simulink model "uvod_PID"  (R2023a)
settings: Solver=VariableStepAuto  StartTime=0.0  StopTime=40  RelTol=1e-3
values from neighbouring files (symbols this model uses):
  T = 0.01    [D1.m]    (also in D1_param.m)
libraries: simulink x1
settings Model: Creator=rapaja  LastModifiedBy=aleks
settings SolverCC: AlgebraicLoopSolver=TrustRegion
settings DebuggingCC: UnconnectedInputMsg=warning  UnconnectedOutputMsg=warning  UnconnectedLineMsg=warning
settings ModelReferenceCC: EnableRefExpFcnMdlSchedulingChecks=on

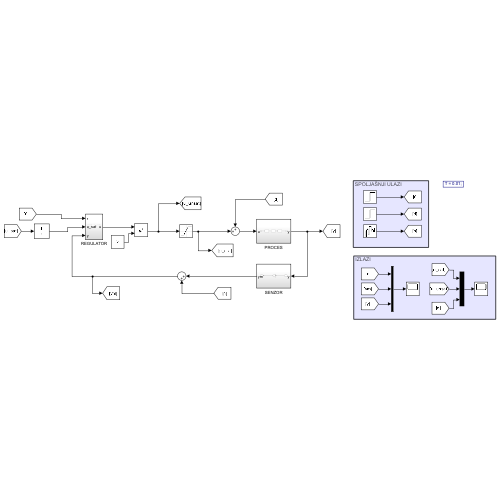
[thumbnail: Simulink's stored preview of the top-level diagram]
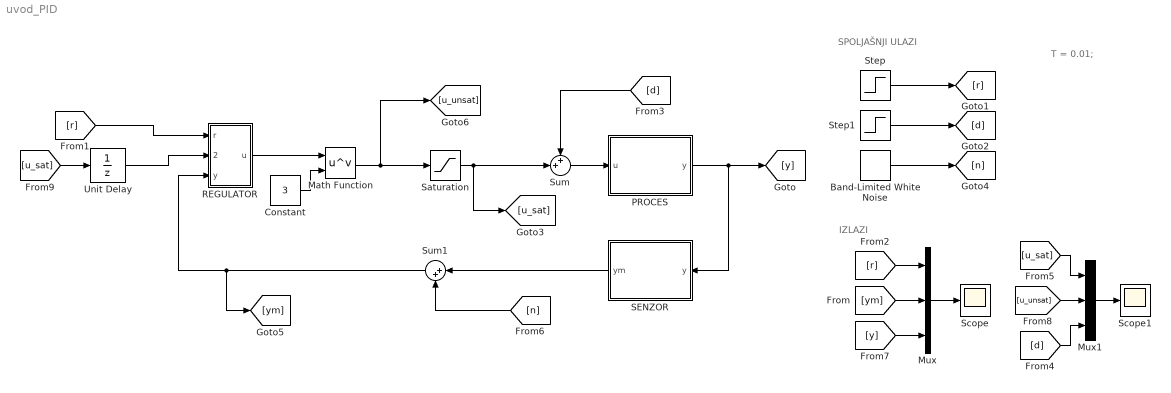
== system uvod_PID ==
  note: T = 0.01;
  note: IZLAZI
  note: SPOLJAŠNJI ULAZI
  Band-Limited White Noise : simulink/Sources/Band-Limited White Noise  Cov=[0.00001]  Ts=T  seed=[23341]
  Constant : Constant  Value=3
  Math Function : Math  Operator=pow
  Mux : Mux  Inputs=3
  Mux1 : Mux  Inputs=3
  PROCES : Subsystem
  REGULATOR : Subsystem
  SENZOR : Subsystem
  Saturation : Saturate  UpperLimit=1  LowerLimit=-1
  Scope : Scope
  Scope1 : Scope
  Step : Step  SampleTime=0
  Step1 : Step  Time=10  SampleTime=0
  Sum : Sum  Inputs=++|
  Sum1 : Sum  Inputs=|++
  Unit Delay : UnitDelay  SampleTime=-1  HasFrameUpgradeWarning=on
  wires:
  [r] -> Mux/1
  [ym] -> Mux/2
  Mux/1 -> Scope/1
  Step/1 -> [r]
  Sum/1 -> PROCES/1(u)
  PROCES/1(y) -> [y], SENZOR/1(y)
  [r] -> REGULATOR/1(r)
  Sum1/1 -> [ym], REGULATOR/3(y)
  Mux1/1 -> Scope1/1
  [d] -> Mux1/3
  [u_sat] -> Mux1/1
  SENZOR/1(ym) -> Sum1/1
  Band-Limited White Noise/1 -> [n]
  [n] -> Sum1/2
  [y] -> Mux/3
  [d] -> Sum/1
  REGULATOR/1(u) -> Math Function/1
  Saturation/1 -> [u_sat], Sum/2
  [u_unsat] -> Mux1/2
  [u_sat] -> Unit Delay/1
  Unit Delay/1 -> REGULATOR/2(u_sat)
  Step1/1 -> [d]
  Math Function/1 -> [u_unsat], Saturation/1
  Constant/1 -> Math Function/2

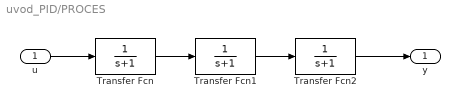
== system uvod_PID/PROCES ==
  u : Inport
  Transfer Fcn : TransferFcn  Denominator=[1 1]
  Transfer Fcn1 : TransferFcn  Denominator=[1 1]
  Transfer Fcn2 : TransferFcn  Denominator=[1 1]
  y : Outport
  wires:
  Transfer Fcn/1 -> Transfer Fcn1/1
  Transfer Fcn1/1 -> Transfer Fcn2/1
  u/1 -> Transfer Fcn/1
  Transfer Fcn2/1 -> y/1

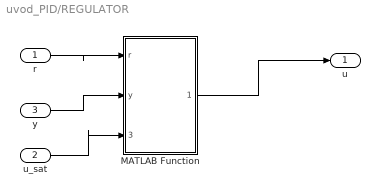
== system uvod_PID/REGULATOR ==
  r : Inport
  u_sat : Inport  Port=2
  y : Inport  Port=3
  MATLAB Function : MATLAB Function  TreatAsAtomicUnit=on
  u : Outport
  wires:
  r/1 -> MATLAB Function/1(r)
  y/1 -> MATLAB Function/2(y)
  MATLAB Function/1(u_unsat) -> u/1
  u_sat/1 -> MATLAB Function/3(u_sat_prev)

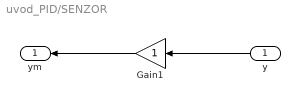
== system uvod_PID/SENZOR ==
  y : Inport
  Gain1 : Gain
  ym : Outport
  wires:
  y/1 -> Gain1/1
  Gain1/1 -> ym/1

== matlab function uvod_PID/REGULATOR/MATLAB Function ==
  settings: updateMethod=DISCRETE
  data: r input; u_unsat output; y input; u_sat_prev input
function u_unsat = PID_regulator(r, y, u_sat_prev)

Kp = 3.7;
Ki = 2.5;
Kd = 2.2;
Ts = 0.01;

N = 10;
Kaw = 1/Kp;

persistent I y_prev D_prev u_unsat_prev
if isempty(I)
    I = 0;
    y_prev = 0;
    D_prev = 0;
    u_unsat_prev = 0;
end

e = r - y;

if nargin >= 3 && ~isempty(u_sat_prev)
    sat_error = u_sat_prev - u_unsat_prev;
    I = I + Kaw * sat_error;
end

D_unfilt = -(y - y_prev) / Ts;
alpha = N * Ts / (1 + N * Ts);
D = alpha * D_unfilt + (1 - alpha) * D_prev;

P = Kp * e;
D_term = Kd * D;
I = I + Ki * Ts * e;

u_unsat = P + I + D_term;

y_prev = y;
D_prev = D;
u_unsat_prev = u_unsat;

end
